simulink model "mpu_imu"  (R2015b)
settings: Solver=ode5  StartTime=0.0  StopTime=250  FixedStep=1/mpu_sampling_frequency  RelTol=1e-3
values from neighbouring files (symbols this model uses):
  mpu_ax_noise_density = 300e-6    (= 0.0003)    [imu_settings.m]    (also in mpu_ax.m)
  mpu_ax_sensitivity = 1/16384    (= 6.103515625e-05)    [imu_settings.m]    (also in mpu_ax.m)
  mpu_ax_w = 460    [imu_settings.m]    (also in mpu_ax.m)
  mpu_gyro_noise_density = 0.01    [imu_settings.m]    (also in mpu_plot.m)
  mpu_gyro_sensitivity = 0.0610    (= 0.061)    [imu_settings.m]    (also in mpu_plot.m)
  mpu_sampling_frequency = 819.2    [adis_imu_settings.m]    (also in imu_settings.m = 200; mpu_plot.m = 200)
  mpu_w = 250    [imu_settings.m]    (also in mpu_plot.m)
  wn = gyroscope_wn    (= 17500)    [PrepCode.m]
  zeta = 0.5    [PrepCode.m]
undefined symbols (not defined in the file or in its folder): DiscIntNeverNeededParam, w_ax, wn_ax, zeta_ax
libraries: simulink x6, vrlib x2
settings Model: Creator=TOOsab  LastModifiedBy=TOOsab

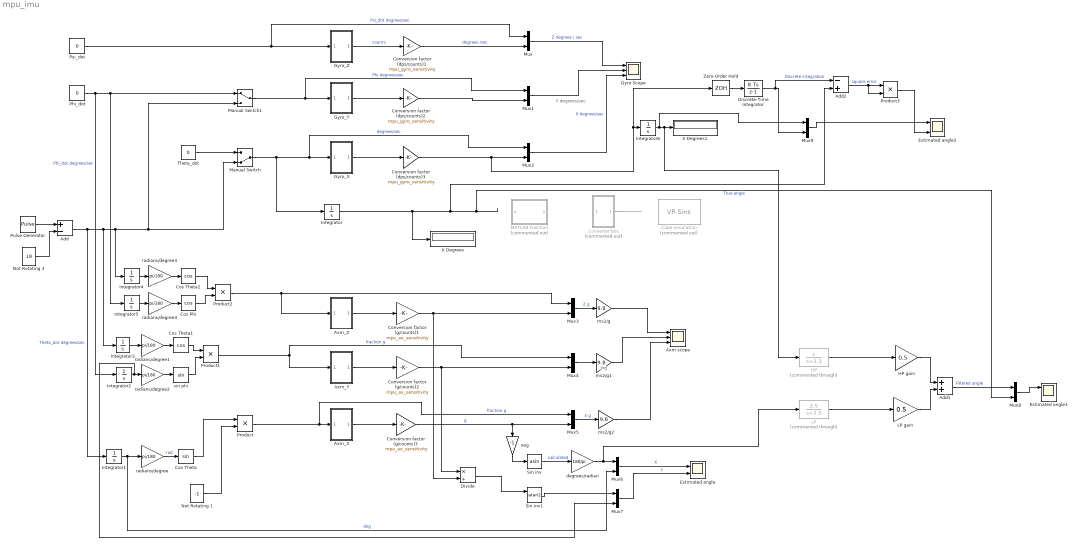
== system mpu_imu ==
  note: Y degrees/sec
  note: Y g
  Add : Sum  Inputs=+-
  Add1 : Sum
  Add2 : Sum  Inputs=-+
  Axm scope : Scope  NumInputPorts=3
  Axm_X : Subsystem
  Axm_Y : Subsystem
  Axm_Z : Subsystem
  Conversion factor (dps/counts)1 : Gain  Gain=mpu_gyro_sensitivity
  Conversion factor (dps/counts)2 : Gain  Gain=mpu_gyro_sensitivity
  Conversion factor (dps/counts)3 : Gain  Gain=mpu_gyro_sensitivity
  Conversion factor (g/counts)1 : Gain  Gain=mpu_ax_sensitivity
  Conversion factor (g/counts)2 : Gain  Gain=mpu_ax_sensitivity
  Conversion factor (g/counts)3 : Gain  Gain=mpu_ax_sensitivity
  Converter box : Subsystem  Commented=on
  Cos Phi : Trigonometry  Operator=cos
  Cos Theta : Trigonometry
  Cos Theta1 : Trigonometry  Operator=cos
  Cos Theta2 : Trigonometry  Operator=cos
  Cube simulation : vrlib/VR Sink  Commented=on  InstantiateOnLoad=on  SampleTime=0.1  ViewEnable=on  RemoteChange=off  RemoteView=off  FieldsWritten=B1.rotation.4.1.1.double  WorldFileName=C:\Users\TOOsab\Documents\MATLAB\boxv2.0.wrl  WorldDescription=box2  AutoView=on  VideoDimensions=[]  AllowVariableSize=off  FigureProperties="{'Position', 'Name', 'Viewpoint', 'CameraBound', 'CameraDirection', 'CameraPosition', 'CameraUpVector', 'ZoomFactor', 'Antialiasing', 'Headlight', 'Lighting', 'NavPanel', 'Sound', 'StatusBar', 'Stereo3D', 'Stereo3DCameraOffset', 'Stereo3DHIT', 'ToolBar', 'Textures', 'Transparency', 'Triad', 'Wireframe', 'NavZones', 'NavMode', 'NavSpeed', 'CaptureFileFormat', 'CaptureFileName', 'Record2DCompressMethod', 'Record2DCompressQuality', 'Record2D', 'Record2DFileName', 'Record2DFPS'; [5.0000000000000000e+00   9.2000000000000000e+01   5.7600000000000000e+02   3.8000000000000000e+02], 'box2', '', 'on', [2.1122870184322479e-01   0.0000000000000000e+00  -9.7743666573217214e-01], [-1.3610137701034546e+00   0.0000000000000000e+00   8.6030883789062500e+00], [0.0000000000000000e+00   1.0000000000000000e+00   0.0000000000000000e+00], [1.0000000000000000e+00], 'on', 'on', 'on', 'halfbar', 'on', 'on', 'off', [1.0000000149011612e-01], [0.0000000000000000e+00], 'on', 'on', 'on', 'none', 'on', 'off', 'walk', 'normal', 'tif', '%f_anim_%n.tif', 'auto', [7.5000000000000000e+01], 'off', '%f_anim_%n.avi', 'auto'}"
  Discrete-Time Integrator : DiscreteIntegrator  InitialConditionSetting=State (most efficient)  SampleTime=-1  ICPrevOutput=DiscIntNeverNeededParam  ICPrevScaledInput=DiscIntNeverNeededParam
  Divide : Product  Inputs=*/
  Estimated angle : Scope  NumInputPorts=2
  Estimated angle1 : Scope  NumInputPorts=2
  Estimated angle2 : Scope  NumInputPorts=2
  Gyro Scope : Scope  NumInputPorts=3
  Gyro_X : Subsystem
  Gyro_Y : Subsystem
  Gyro_Z : Subsystem
  HP : TransferFcn  Commented=through  Numerator=[1 0]  Denominator=[1 3.3]
  HP gain : Gain  Gain=0.5
  Integrator{,1..6} (7 alike) : Integrator
  LP : TransferFcn  Commented=through  Numerator=[2.5]  Denominator=[1 2.5]
  LP gain : Gain  Gain=0.5
  MATLAB Function : MATLAB Function  Commented=on  TreatAsAtomicUnit=on
  Manual Switch : ManualSwitch  CurrentSetting=0
  Manual Switch1 : ManualSwitch
  Mux{,1..8} (9 alike) : Mux  Inputs=2
  Mux9 : Mux  Inputs=3
  Not Rotating 1 : Constant  Value=-1
  Not Rotating 3 : Constant  Value=18
  Phi_dot : Constant  Value=0
  Product{,1..3} (4 alike) : Product
  Psi_dot : Constant  Value=0
  Pulse Generator : DiscretePulseGenerator  PulseType=Time based  Amplitude=36  Period=50  PulseWidth=50
  Sin inv : Trigonometry  Operator=asin
  Sin inv1 : Trigonometry  Operator=atan2
  Theta_dot : Constant  Value=0
  X Degrees : Display
  X Degrees1 : Display
  Zero-Order Hold : ZeroOrderHold  SampleTime=1/mpu_sampling_frequency
  degrees/radian : Gain  Gain=180/pi
  ms2/g : Gain  Gain=9.8
  ms2/g1 : Gain  Gain=9.8
  ms2/g2 : Gain  Gain=9.8
  neg : Gain  Gain=-1
  radians/degree{,1..4} (5 alike) : Gain  Gain=pi/180
  sin phi : Trigonometry
  wires:
  Gyro_Z/1(Out1) -> Conversion factor (dps/counts)1/1  "counts"
  Manual Switch1/1 -> Gyro_Y/1(In1), Mux1/1  "Phi degrees/sec"
  Manual Switch/1 -> Integrator/1, Mux2/1, Gyro_X/1(In1)  "degrees/sec"
  Gyro_Y/1(Out1) -> Conversion factor (dps/counts)2/1
  Gyro_X/1(Out1) -> Conversion factor (dps/counts)3/1
  Conversion factor (dps/counts)1/1 -> Mux/2  "degrees /sec"
  Conversion factor (dps/counts)2/1 -> Mux1/2
  Conversion factor (dps/counts)3/1 -> Zero-Order Hold/1, Integrator6/1, Mux2/2
  Mux/1 -> Gyro Scope/1  "Z degrees / sec"
  Mux1/1 -> Gyro Scope/2
  Mux2/1 -> Gyro Scope/3  "X degrees/sec"
  Psi_dot/1 -> Mux/1, Gyro_Z/1(In1)  "Psi_dot degrees/sec"
  Theta_dot/1 -> Manual Switch/1
  Phi_dot/1 -> Integrator2/1, Integrator5/1, Manual Switch1/1  "Phi_dot degrees/sec"
  Product2/1 -> Mux3/1, Axm_Z/1(In1)
  Axm_Z/1(Out1) -> Conversion factor (g/counts)1/1
  Mux3/1 -> ms2/g/1  "Z g"
  Mux4/1 -> ms2/g1/1
  Mux5/1 -> ms2/g2/1  "X g"
  Product1/1 -> Axm_Y/1(In1), Mux4/1  "fraction g"
  Axm_Y/1(Out1) -> Conversion factor (g/counts)2/1
  Conversion factor (g/counts)2/1 -> Divide/1, Mux4/2
  Axm_X/1(Out1) -> Conversion factor (g/counts)3/1
  Conversion factor (g/counts)3/1 -> Mux5/2, neg/1  "g"
  ms2/g/1 -> Axm scope/1
  ms2/g1/1 -> Axm scope/2
  ms2/g2/1 -> Axm scope/3
  Integrator/1 -> Add2/2, Mux8/2, X Degrees/1  "True angle"
  Pulse Generator/1 -> Add/1
  Add/1 -> Integrator1/1, Integrator3/1, Integrator4/1, Manual Switch1/2, Manual Switch/2  "Theta_dot degrees/sec"
  Not Rotating 3/1 -> Add/2
  Cos Theta/1 -> Product/1
  Product/1 -> Mux5/1, Axm_X/1(In1)  "fraction g"
  Not Rotating 1/1 -> Product/2
  Integrator1/1 -> Mux6/2, radians/degree/1  "deg"
  radians/degree/1 -> Cos Theta/1  "rad"
  Integrator3/1 -> radians/degree1/1
  Integrator2/1 -> Mux7/2, radians/degree2/1
  radians/degree1/1 -> Cos Theta1/1
  radians/degree2/1 -> sin phi/1
  Integrator4/1 -> radians/degree3/1
  radians/degree3/1 -> Cos Theta2/1
  Cos Theta1/1 -> Product1/1
  sin phi/1 -> Product1/2
  Cos Theta2/1 -> Product2/1
  Integrator5/1 -> radians/degree4/1
  radians/degree4/1 -> Cos Phi/1
  Cos Phi/1 -> Product2/2
  ? -> Converter box/1(In1)
  Converter box/1(Out1) -> ?
  Sin inv/1 -> degrees/radian/1  "calculated"
  Mux6/1 -> Estimated angle/1  "X"
  degrees/radian/1 -> LP/1, Mux6/1
  neg/1 -> Sin inv/1
  Divide/1 -> Sin inv1/1
  Sin inv1/1 -> Mux7/1
  Mux7/1 -> Estimated angle/2  "Y"
  Integrator6/1 -> Mux9/1, HP/1, X Degrees1/1
  HP gain/1 -> Add1/1
  HP/1 -> HP gain/1
  LP gain/1 -> Add1/2
  LP/1 -> LP gain/1
  Add1/1 -> Mux8/1  "Filtered angle"
  Mux8/1 -> Estimated angle1/1
  Conversion factor (g/counts)1/1 -> Divide/2, Mux3/2
  Mux9/1 -> Estimated angle2/1
  Zero-Order Hold/1 -> Discrete-Time Integrator/1
  Discrete-Time Integrator/1 -> Add2/1, Mux9/3  "Discrete integration"
  Add2/1 -> Product3/2, Product3/1  "square error"
  Product3/1 -> Estimated angle2/2

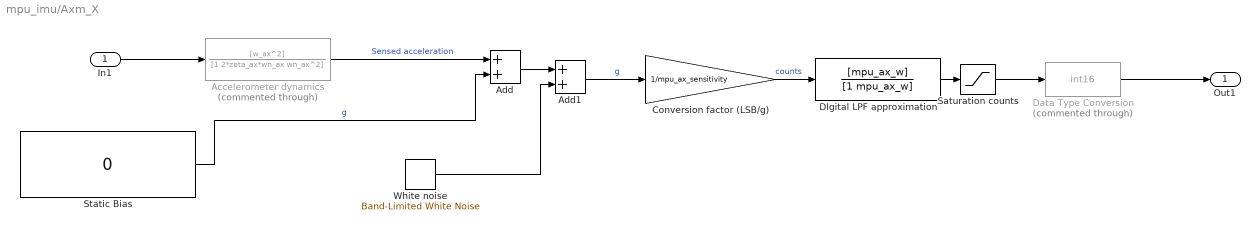
== system mpu_imu/Axm_X ==
  In1 : Inport
  Accelerometer dynamics : TransferFcn  Commented=through  Numerator=[w_ax^2]  Denominator=[1 2*zeta_ax*wn_ax wn_ax^2]
  Add : Sum
  Add1 : Sum
  Conversion factor (LSB/g) : Gain  Gain=1/mpu_ax_sensitivity
  DIgital LPF approximation : TransferFcn  Numerator=[mpu_ax_w]  Denominator=[1 mpu_ax_w]
  Data Type Conversion : DataTypeConversion  Commented=through  OutDataTypeStr=int16
  "Saturation counts " : Saturate  UpperLimit=2^15  LowerLimit=-2^15
  Static Bias : Constant  Value=0
  White noise : simulink/Sources/Band-Limited White Noise  Cov=[(mpu_ax_noise_density)^2]  Ts=1/mpu_sampling_frequency  seed=[23341]
  Out1 : Outport
  wires:
  In1/1 -> Accelerometer dynamics/1
  Data Type Conversion/1 -> Out1/1
  "Saturation counts "/1 -> Data Type Conversion/1
  DIgital LPF approximation/1 -> "Saturation counts "/1
  Add1/1 -> Conversion factor (LSB/g)/1  "g"
  Add/1 -> Add1/1
  White noise/1 -> Add1/2
  Accelerometer dynamics/1 -> Add/1  "Sensed acceleration"
  Static Bias/1 -> Add/2  "g"
  Conversion factor (LSB/g)/1 -> DIgital LPF approximation/1  "counts"

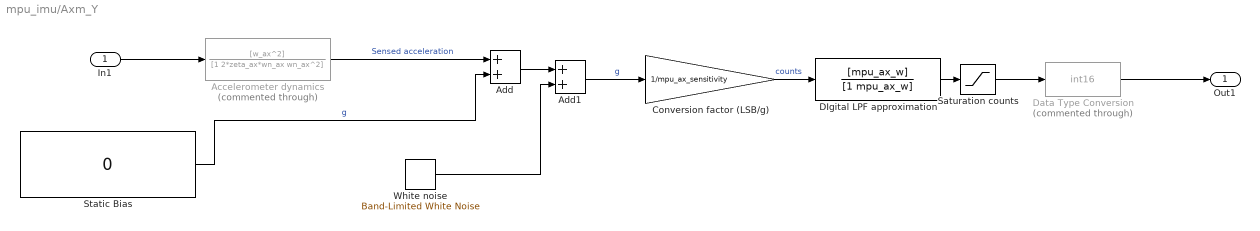
== system mpu_imu/Axm_Y ==
  In1 : Inport
  Accelerometer dynamics : TransferFcn  Commented=through  Numerator=[w_ax^2]  Denominator=[1 2*zeta_ax*wn_ax wn_ax^2]
  Add : Sum
  Add1 : Sum
  Conversion factor (LSB/g) : Gain  Gain=1/mpu_ax_sensitivity
  DIgital LPF approximation : TransferFcn  Numerator=[mpu_ax_w]  Denominator=[1 mpu_ax_w]
  Data Type Conversion : DataTypeConversion  Commented=through  OutDataTypeStr=int16
  "Saturation counts " : Saturate  UpperLimit=2^15  LowerLimit=-2^15
  Static Bias : Constant  Value=0
  White noise : simulink/Sources/Band-Limited White Noise  Cov=[(mpu_ax_noise_density)^2]  Ts=1/mpu_sampling_frequency  seed=[23341]
  Out1 : Outport
  wires:
  In1/1 -> Accelerometer dynamics/1
  Data Type Conversion/1 -> Out1/1
  "Saturation counts "/1 -> Data Type Conversion/1
  DIgital LPF approximation/1 -> "Saturation counts "/1
  Add1/1 -> Conversion factor (LSB/g)/1  "g"
  Add/1 -> Add1/1
  White noise/1 -> Add1/2
  Accelerometer dynamics/1 -> Add/1  "Sensed acceleration"
  Static Bias/1 -> Add/2  "g"
  Conversion factor (LSB/g)/1 -> DIgital LPF approximation/1  "counts"

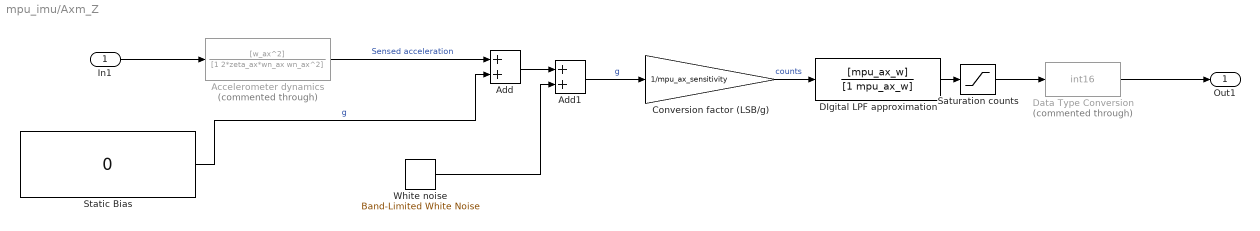
== system mpu_imu/Axm_Z ==
  In1 : Inport
  Accelerometer dynamics : TransferFcn  Commented=through  Numerator=[w_ax^2]  Denominator=[1 2*zeta_ax*wn_ax wn_ax^2]
  Add : Sum
  Add1 : Sum
  Conversion factor (LSB/g) : Gain  Gain=1/mpu_ax_sensitivity
  DIgital LPF approximation : TransferFcn  Numerator=[mpu_ax_w]  Denominator=[1 mpu_ax_w]
  Data Type Conversion : DataTypeConversion  Commented=through  OutDataTypeStr=int16
  "Saturation counts " : Saturate  UpperLimit=2^15  LowerLimit=-2^15
  Static Bias : Constant  Value=0
  White noise : simulink/Sources/Band-Limited White Noise  Cov=[(mpu_ax_noise_density)^2]  Ts=1/mpu_sampling_frequency  seed=[23341]
  Out1 : Outport
  wires:
  In1/1 -> Accelerometer dynamics/1
  Data Type Conversion/1 -> Out1/1
  "Saturation counts "/1 -> Data Type Conversion/1
  DIgital LPF approximation/1 -> "Saturation counts "/1
  Add1/1 -> Conversion factor (LSB/g)/1  "g"
  Add/1 -> Add1/1
  White noise/1 -> Add1/2
  Accelerometer dynamics/1 -> Add/1  "Sensed acceleration"
  Static Bias/1 -> Add/2  "g"
  Conversion factor (LSB/g)/1 -> DIgital LPF approximation/1  "counts"

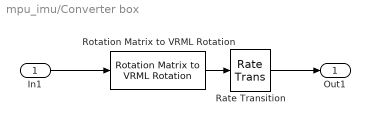
== system mpu_imu/Converter box ==
  In1 : Inport
  Rate Transition : RateTransition
  Rotation Matrix to VRML Rotation : vrlib/Utilities/Rotation Matrix to VRML Rotation  maxzero=1e-12
  Out1 : Outport
  wires:
  In1/1 -> Rotation Matrix to VRML Rotation/1
  Rotation Matrix to VRML Rotation/1 -> Rate Transition/1
  Rate Transition/1 -> Out1/1

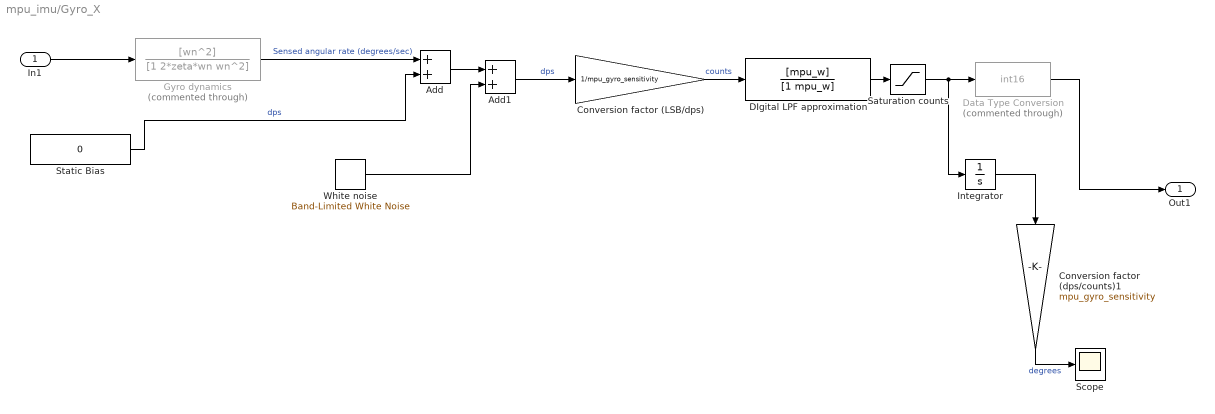
== system mpu_imu/Gyro_X ==
  In1 : Inport
  Add : Sum
  Add1 : Sum
  Conversion factor (LSB/dps) : Gain  Gain=1/mpu_gyro_sensitivity
  Conversion factor (dps/counts)1 : Gain  Gain=mpu_gyro_sensitivity
  DIgital LPF approximation : TransferFcn  Numerator=[mpu_w]  Denominator=[1 mpu_w]
  Data Type Conversion : DataTypeConversion  Commented=through  OutDataTypeStr=int16
  Gyro dynamics : TransferFcn  Commented=through  Numerator=[wn^2]  Denominator=[1 2*zeta*wn wn^2]
  Integrator : Integrator
  "Saturation counts " : Saturate  UpperLimit=2^15  LowerLimit=-2^15
  Scope : Scope
  Static Bias : Constant  Value=0
  White noise : simulink/Sources/Band-Limited White Noise  Cov=[(mpu_gyro_noise_density)^2]  Ts=1/mpu_sampling_frequency  seed=[23341]
  Out1 : Outport
  wires:
  Gyro dynamics/1 -> Add/1  "Sensed angular rate (degrees/sec)"
  White noise/1 -> Add1/2
  Static Bias/1 -> Add/2  "dps"
  Conversion factor (LSB/dps)/1 -> DIgital LPF approximation/1  "counts"
  Add/1 -> Add1/1
  Conversion factor (dps/counts)1/1 -> Scope/1  "degrees"
  Integrator/1 -> Conversion factor (dps/counts)1/1
  Data Type Conversion/1 -> Out1/1
  In1/1 -> Gyro dynamics/1
  "Saturation counts "/1 -> Integrator/1, Data Type Conversion/1
  DIgital LPF approximation/1 -> "Saturation counts "/1
  Add1/1 -> Conversion factor (LSB/dps)/1  "dps"

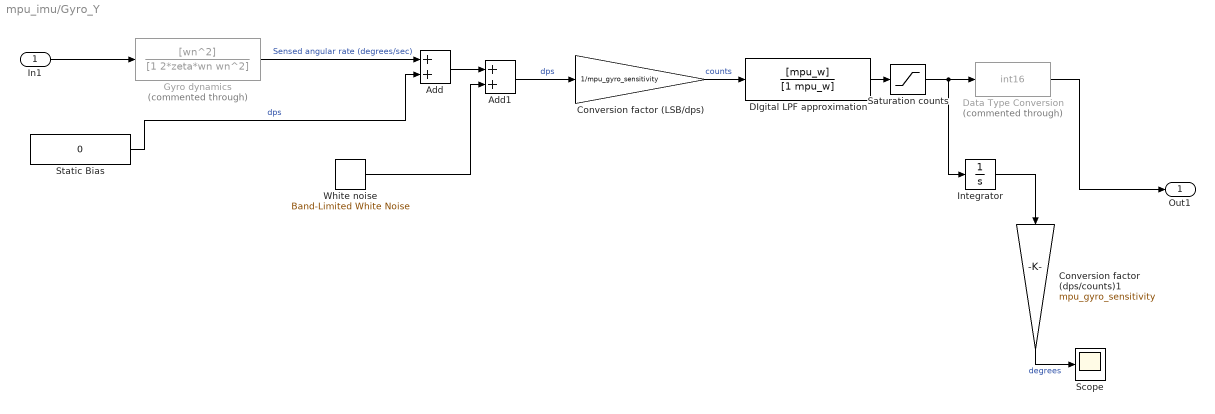
== system mpu_imu/Gyro_Y ==
  In1 : Inport
  Add : Sum
  Add1 : Sum
  Conversion factor (LSB/dps) : Gain  Gain=1/mpu_gyro_sensitivity
  Conversion factor (dps/counts)1 : Gain  Gain=mpu_gyro_sensitivity
  DIgital LPF approximation : TransferFcn  Numerator=[mpu_w]  Denominator=[1 mpu_w]
  Data Type Conversion : DataTypeConversion  Commented=through  OutDataTypeStr=int16
  Gyro dynamics : TransferFcn  Commented=through  Numerator=[wn^2]  Denominator=[1 2*zeta*wn wn^2]
  Integrator : Integrator
  "Saturation counts " : Saturate  UpperLimit=2^15  LowerLimit=-2^15
  Scope : Scope
  Static Bias : Constant  Value=0
  White noise : simulink/Sources/Band-Limited White Noise  Cov=[(mpu_gyro_noise_density)^2]  Ts=1/mpu_sampling_frequency  seed=[23341]
  Out1 : Outport
  wires:
  Add1/1 -> Conversion factor (LSB/dps)/1  "dps"
  DIgital LPF approximation/1 -> "Saturation counts "/1
  "Saturation counts "/1 -> Data Type Conversion/1, Integrator/1
  In1/1 -> Gyro dynamics/1
  Data Type Conversion/1 -> Out1/1
  Integrator/1 -> Conversion factor (dps/counts)1/1
  Conversion factor (dps/counts)1/1 -> Scope/1  "degrees"
  Add/1 -> Add1/1
  Conversion factor (LSB/dps)/1 -> DIgital LPF approximation/1  "counts"
  Static Bias/1 -> Add/2  "dps"
  White noise/1 -> Add1/2
  Gyro dynamics/1 -> Add/1  "Sensed angular rate (degrees/sec)"

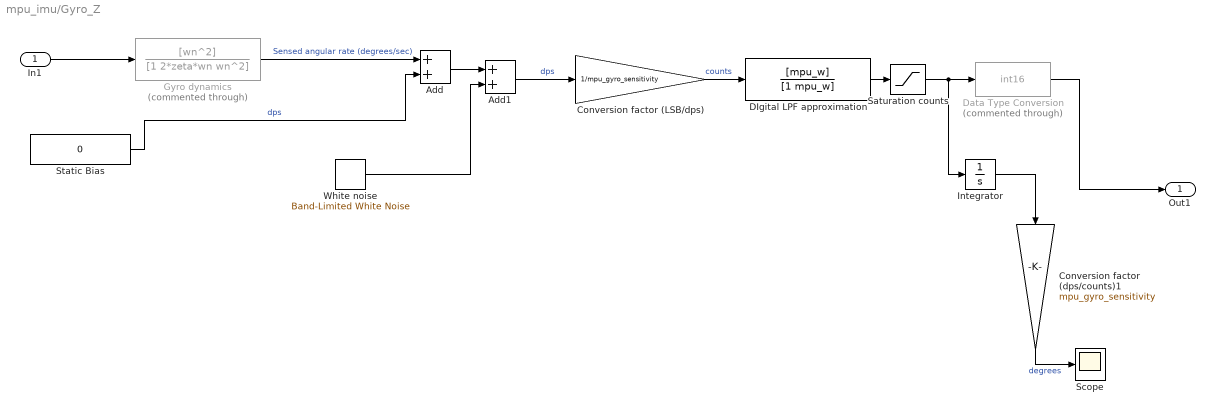
== system mpu_imu/Gyro_Z ==
  In1 : Inport
  Add : Sum
  Add1 : Sum
  Conversion factor (LSB/dps) : Gain  Gain=1/mpu_gyro_sensitivity
  Conversion factor (dps/counts)1 : Gain  Gain=mpu_gyro_sensitivity
  DIgital LPF approximation : TransferFcn  Numerator=[mpu_w]  Denominator=[1 mpu_w]
  Data Type Conversion : DataTypeConversion  Commented=through  OutDataTypeStr=int16
  Gyro dynamics : TransferFcn  Commented=through  Numerator=[wn^2]  Denominator=[1 2*zeta*wn wn^2]
  Integrator : Integrator
  "Saturation counts " : Saturate  UpperLimit=2^15  LowerLimit=-2^15
  Scope : Scope
  Static Bias : Constant  Value=0
  White noise : simulink/Sources/Band-Limited White Noise  Cov=[(mpu_gyro_noise_density)^2]  Ts=1/mpu_sampling_frequency  seed=[23341]
  Out1 : Outport
  wires:
  Gyro dynamics/1 -> Add/1  "Sensed angular rate (degrees/sec)"
  White noise/1 -> Add1/2
  Static Bias/1 -> Add/2  "dps"
  Conversion factor (LSB/dps)/1 -> DIgital LPF approximation/1  "counts"
  Add/1 -> Add1/1
  Conversion factor (dps/counts)1/1 -> Scope/1  "degrees"
  Integrator/1 -> Conversion factor (dps/counts)1/1
  Data Type Conversion/1 -> Out1/1
  In1/1 -> Gyro dynamics/1
  "Saturation counts "/1 -> Integrator/1, Data Type Conversion/1
  DIgital LPF approximation/1 -> "Saturation counts "/1
  Add1/1 -> Conversion factor (LSB/dps)/1  "dps"

== matlab function mpu_imu/MATLAB Function ==
  data: u input; y output
function y = fcn(u)
%#codegen

y = rotx(u);
